simulink model "RLC"  (Simulink 7.1)
settings: Solver=ode45  StartTime=0.0  StopTime=.03  RelTol=1e-3
undefined symbols (not defined in the file): C, L, R, V
settings Model: Creator=Smrit  LastModifiedBy=Smrit

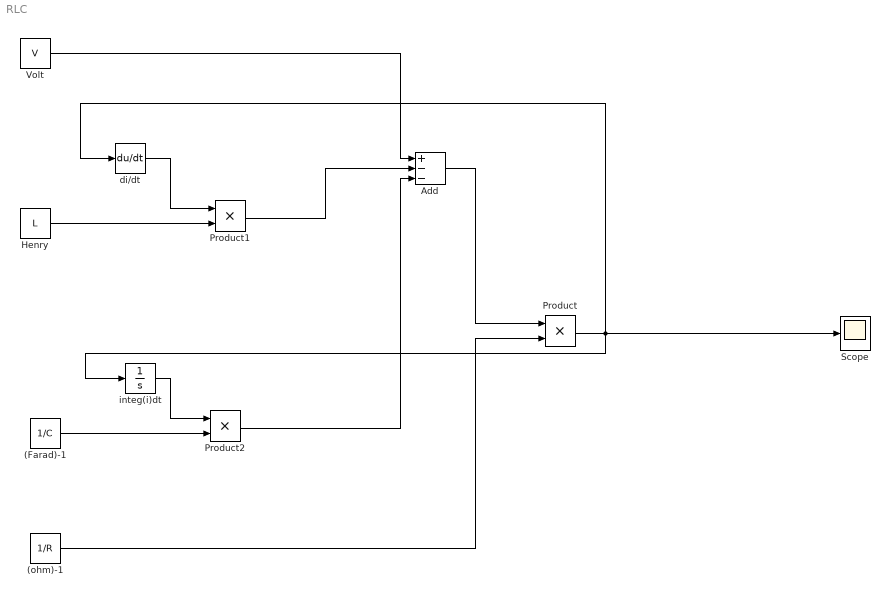
== system RLC ==
  (Farad)-1 : Constant  Value=1/C  OutDataType=sfix(16)  OutScaling=2^0
  (ohm)-1 : Constant  Value=1/R  OutDataType=sfix(16)  OutScaling=2^0
  Add : Sum  Inputs=+--  OutDataType=sfix(16)  OutScaling=2^-10
  Henry : Constant  Value=L  OutDataType=sfix(16)  OutScaling=2^0
  Product : Product  OutDataType=sfix(16)  OutScaling=2^0  RndMeth=Zero
  Product1 : Product  OutDataType=sfix(16)  OutScaling=2^0  RndMeth=Zero
  Product2 : Product  OutDataType=sfix(16)  OutScaling=2^0  RndMeth=Zero
  Scope : Scope
  Volt : Constant  Value=V  OutDataType=sfix(16)  OutScaling=2^0
  di/dt : Derivative
  integ(i)dt : Integrator
  wires:
  di/dt/1 -> Product1/1
  Henry/1 -> Product1/2
  Volt/1 -> Add/1
  Product1/1 -> Add/2
  integ(i)dt/1 -> Product2/1
  (Farad)-1/1 -> Product2/2
  Product2/1 -> Add/3
  Add/1 -> Product/1
  (ohm)-1/1 -> Product/2
  Product/1 -> Scope/1, di/dt/1, integ(i)dt/1
